simulink model "SL7_2_13"  (R2015b)
settings: Solver=VariableStepAuto  StartTime=0.0  StopTime=10.0  RelTol=1e-3
settings Model: Creator=Administrator  LastModifiedBy=Administrator

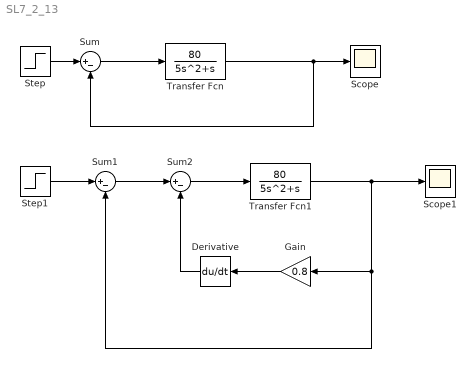
== system SL7_2_13 ==
  Derivative : Derivative
  Gain : Gain  Gain=0.8
  Scope : Scope
  Scope1 : Scope
  Step : Step  Time=0  SampleTime=0
  Step1 : Step  Time=0  SampleTime=0
  Sum : Sum  Inputs=|+-
  Sum1 : Sum  Inputs=|+-
  Sum2 : Sum  Inputs=|+-
  Transfer Fcn : TransferFcn  Numerator=[80]  Denominator=[5 1 0]
  Transfer Fcn1 : TransferFcn  Numerator=[80]  Denominator=[5 1 0]
  wires:
  Transfer Fcn/1 -> Sum/2, Scope/1
  Step/1 -> Sum/1
  Transfer Fcn1/1 -> Gain/1, Sum1/2, Scope1/1
  Step1/1 -> Sum1/1
  Sum/1 -> Transfer Fcn/1
  Sum2/1 -> Transfer Fcn1/1
  Sum1/1 -> Sum2/1
  Derivative/1 -> Sum2/2
  Gain/1 -> Derivative/1
